simulink model "fluid_animated"  (Simulink 6.0)
settings: Solver=ode45  StartTime=0.0  StopTime=50.0  MaxStep=0.01  RelTol=1e-3
values from neighbouring files (symbols this model uses):
  A = [(-1*(1/(C1*R1)+1/(C1*R2)))    1/(C1*R2)                   0 ... (first row only)    [fluid_animation_init.m]
  B = [1/(C1*R1); 0; 0]    [fluid_animation_init.m]
  C = [eye(3,3)*1/(rho*g) ... (first row only)    [fluid_animation_init.m]    (also in tank_capacitance.m = A/rho/g)
  D = zeros(m,1)    [fluid_animation_init.m]
  g = 9.8    [fluid_animation_init.m]
  omega_0 = 5.45    [fluid_animation_init.m]
  rho = 1000    [fluid_animation_init.m]
  Xo = 0*rho*g*ones(n,1)/2    [fluid_animation_init.m]
undefined symbols (not defined in the file or in its folder): animate_fluid_tank
settings Model: LastModifiedBy=farrell

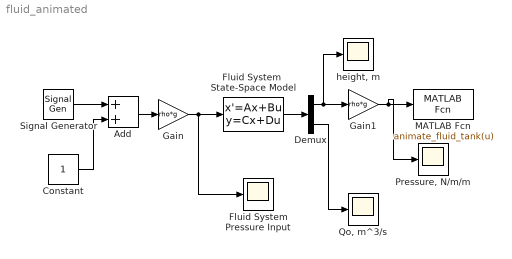
== system fluid_animated ==
  Add : Sum  OutScaling=2^-10
  Constant : Constant
  Demux : Demux  Outputs=[3,1]
  Fluid System Pressure Input : Scope
      settings: TimeRange=50  YMin=0  YMax=20000  SaveName=ScopeData2
  Fluid System  State-Space Model : StateSpace  A=A  B=B  C=C  D=D  X0=Xo
  Gain : Gain  Gain=rho*g
  Gain1 : Gain  Gain=rho*g
  MATLAB Fcn : MATLABFcn  MATLABFcn=animate_fluid_tank(u)  SampleTime=0.01
  "Pressure, N/m/m" : Scope
      settings: TimeRange=50  YMin=0  YMax=14000
  "Qo, m^3/s" : Scope
      settings: TimeRange=50  YMin=0  YMax=0.04  SaveName=ScopeData3
  Signal Generator : SignalGenerator  Frequency=omega_0  Units=rad/sec
  "height, m" : Scope
      settings: TimeRange=50  YMin=0  YMax=1.5
  wires:
  Add/1 -> Gain/1
  Constant/1 -> Add/2
  Signal Generator/1 -> Add/1
  Fluid System  State-Space Model/1 -> Demux/1
  Demux/1 -> "height, m"/1, Gain1/1
  Demux/2 -> "Qo, m^3/s"/1
  Gain/1 -> Fluid System  State-Space Model/1, Fluid System Pressure Input/1
  Gain1/1 -> MATLAB Fcn/1, "Pressure, N/m/m"/1
